simulink model "SHipVar5_OpVnesh"  (R2022a)
settings: Solver=ode23tb  StartTime=0.0  StopTime=time  MaxStep=1e-5  RelTol=1e-5
undefined symbols (not defined in the file): Imax, OpVnesh, Rd, source, U_1
libraries: spsFourierLib x2, spsDiodeLib x1, spsIGBTLib x1, simulink x1, spsSeriesRLCBranchLib x1, spsDCVoltageSourceLib x1, spsVoltageMeasurementLib x1, spsCurrentMeasurementLib x1, spspowerguiLib x1
settings Model: Creator=админ  LastModifiedBy=админ

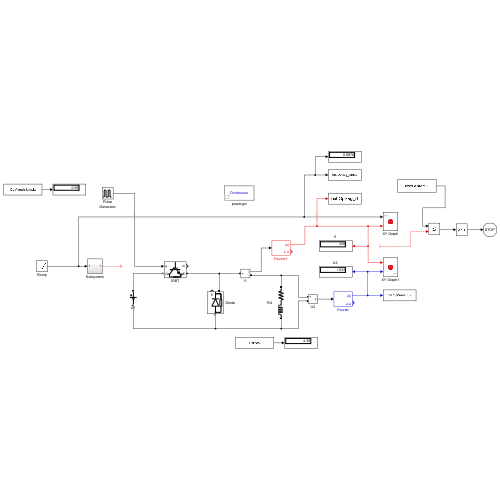
[thumbnail: Simulink's stored preview of the top-level diagram]
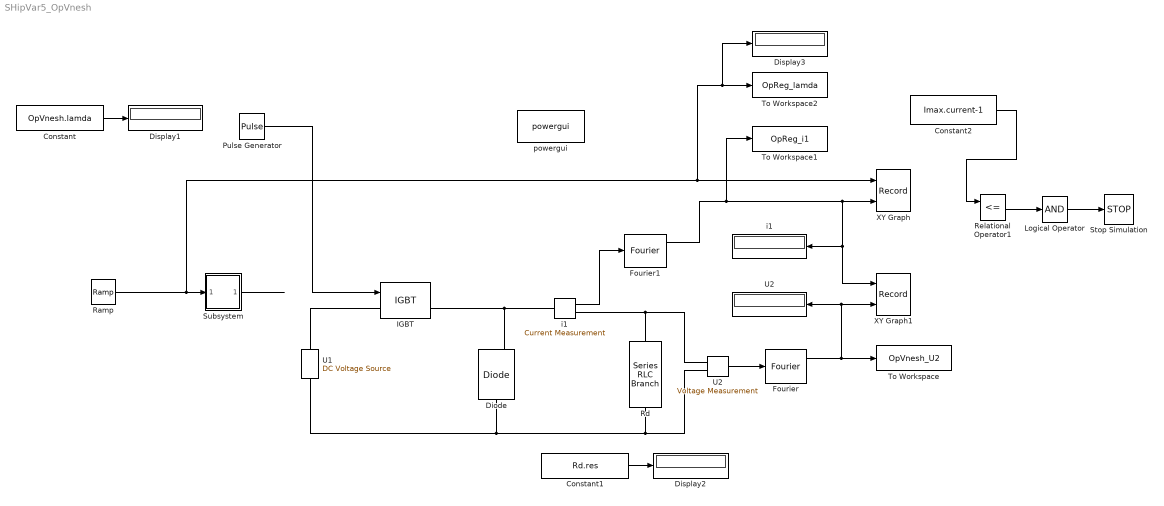
== system SHipVar5_OpVnesh ==
  Constant : Constant  Value=OpVnesh.lamda
  Constant1 : Constant  Value=Rd.res
  Constant2 : Constant  Value=Imax.current-1
  Diode : spsDiodeLib/Diode  Ron=Diode.r_t  Lon=0  Vf=0.8  IC=0  UseSnubber=0  Rs=Diode.R_s  Cs=250e-9  Measurements=on
  Display1 : Display
  Display2 : Display
  Display3 : Display
  Fourier : spsFourierLib/Fourier  Freq=source.f_c  n=0  InInit=[0, 0]  Ts=0
      settings: SourceProductBaseCode=PS
  Fourier1 : spsFourierLib/Fourier  Freq=source.f_c  n=0  InInit=[0, 0]  Ts=0
      settings: SourceProductBaseCode=PS
  IGBT : spsIGBTLib/IGBT  Ron=IGBT.R_on  Lon=0  Vf=IGBT.V_f  Tf=1e-6  Tt=2e-6  IC=0  Rs=1e5  Cs=inf  Measurements=on
  Logical Operator : Logic  Inputs=1  AllPortsSameDT=off  OutDataTypeStr=boolean
  Pulse Generator : DiscretePulseGenerator  PulseType=Time based  Period=1/source.f_c  PulseWidth=OpVnesh.lamda*100
  Ramp : simulink/Sources/Ramp  slope=0.1  start=0  InitialOutput=0
  Rd : spsSeriesRLCBranchLib/Series RLC Branch  LConnTagsString=__new0  RConnTagsString=__new0  BranchType=RL  Resistance=Rd.res  Inductance=Rd.ind  SetiL0=off  InitialCurrent=0  Capacitance=1e-6  Setx0=off  InitialVoltage=0  Measurements=None
  Relational Operator1 : RelationalOperator  Operator=<=  OutDataTypeStr=boolean  RndMeth=Simplest  InputSameDT=off
  Stop Simulation : Stop
  Subsystem : Subsystem
  To Workspace : ToWorkspace  VariableName=OpVnesh_U2  SaveFormat=Structure  SampleTime=-1
      settings: Save2DSignal=2-D array (concatenate along first dimension)
  To Workspace1 : ToWorkspace  VariableName=OpReg_i1  SaveFormat=Structure  SampleTime=-1
      settings: Save2DSignal=2-D array (concatenate along first dimension)
  To Workspace2 : ToWorkspace  VariableName=OpReg_lamda  SaveFormat=Structure  SampleTime=-1
      settings: Save2DSignal=2-D array (concatenate along first dimension)
  U1 : spsDCVoltageSourceLib/DC Voltage Source  Amplitude=U_1  Measurements=None
  U2 : spsVoltageMeasurementLib/Voltage Measurement  PhasorSimulation=off  OutputType=Complex  PSBequivalent=0
  "U2 " : Display
  XY Graph : Record  FileSettingsInternal="{\"entries\":[{\"content\":{\"excelSettings\":{\"content\":{},\"type\":\"Streamout.ExcelSettings\"}},\"type\":\"Streamout.FileSettingStorage\",\"uuid\":\"23574a75-d7b5-437e-9ab1-f31661b62460\"}],\"packageUris\":[\"http://schema.mathworks.com/mf0/streamout_blocks/R2020a\"],\"version\":\"1.0\"}"  Layout=[1 1]  SignalsInternal="{\"entries\":[{\"content\":{\"signals\":[{\"content\":{\"blockPath\":[\"SHipVar5_OpVnesh/XY Graph\"],\"channel\":[],\"dimensions\":[1],\"domain\":\"SHipVar5_OpVnesh/XY Graph\",\"lineColor\":\"#a2142f\",\"plots\":[1],\"port\":1,\"sid\":[\"\"],\"signalID\":4300,\"signalName\":\"Ramp\"},\"type\":\"RecordBlkView.Signal\",\"uuid\":\"330522d2-f3ca-434a-8d93-8c397e8adb3c\"},{\"content\":{\"blockPath\":[\"SHipVar5_OpVnesh/XY Graph\"],\"channel\":[],\"dimensions\":[1],\"domain\":\"SHipVar5_OpVnesh/XY Graph\",\"lineColor\":\"#139fff\",\"plots\":[1],\"port\":2,\"sid\":[\"\"],\"signalID\":4304,\"signalName\":\"Fourier1:1\"},\"type\":\"RecordBlkView.Signal\",\"uuid\":\"7fa0577b-ccd9-48e4-9d98-3b11980c29aa\"}]},\"type\":\"RecordBlkView.InputSignals\",\"uuid\":\"1c9948c1-7f7b-4c40-b817-17e788a1b9c1\"}],\"packageUris\":[\"http://schema.mathworks.com/mf0/streamout_blocks/R2020a\"],\"version\":\"1.0\"}"  VisualizationBindings="{\"xyplotplugin\":{\"info\":[{\"series\":[{\"bindingParametersList\":[{\"parameter\":\"X-Axis\",\"signalID\":4300,\"signalName\":\"Ramp\"},{\"parameter\":\"Y-Axis\",\"signalID\":4304,\"signalName\":\"Fourier1:1\"}],\"seriesID\":45275}],\"subplotID\":1}]}}"  CompatibilityTag=XY
  XY Graph1 : Record  FileSettingsInternal="{\"entries\":[{\"content\":{\"excelSettings\":{\"content\":{},\"type\":\"Streamout.ExcelSettings\"}},\"type\":\"Streamout.FileSettingStorage\",\"uuid\":\"e7ce2358-359a-45fa-9b79-56cba1cac5cb\"}],\"packageUris\":[\"http://schema.mathworks.com/mf0/streamout_blocks/R2020a\"],\"version\":\"1.0\"}"  Layout=[1 1]  SignalsInternal="{\"entries\":[{\"content\":{\"signals\":[{\"content\":{\"blockPath\":[\"SHipVar5_OpVnesh/XY Graph1\"],\"channel\":[],\"dimensions\":[1],\"domain\":\"SHipVar5_OpVnesh/XY Graph1\",\"lineColor\":\"#a2142f\",\"plots\":[1],\"port\":1,\"sid\":[\"\"],\"signalID\":4308,\"signalName\":\"Fourier1:1\"},\"type\":\"RecordBlkView.Signal\",\"uuid\":\"d5f5a975-f57f-42e8-bd8c-c4c1de54bcdc\"},{\"content\":{\"blockPath\":[\"SHipVar5_OpVnesh/XY Graph1\"],\"channel\":[],\"dimensions\":[1],\"domain\":\"SHipVar5_OpVnesh/XY Graph1\",\"lineColor\":\"#139fff\",\"plots\":[1],\"port\":2,\"sid\":[\"\"],\"signalID\":4312,\"signalName\":\"Fourier:1\"},\"type\":\"RecordBlkView.Signal\",\"uuid\":\"1d470808-ef71-43c9-86f4-7795574ddb1a\"}]},\"type\":\"RecordBlkView.InputSignals\",\"uuid\":\"453252bf-c3a8-49dd-a759-dd61e3aad6bf\"}],\"packageUris\":[\"http://schema.mathworks.com/mf0/streamout_blocks/R2020a\"],\"version\":\"1.0\"}"  VisualizationBindings="{\"xyplotplugin\":{\"info\":[{\"series\":[{\"bindingParametersList\":[{\"parameter\":\"X-Axis\",\"signalID\":4308,\"signalName\":\"Fourier1:1\"},{\"parameter\":\"Y-Axis\",\"signalID\":4312,\"signalName\":\"Fourier:1\"}],\"seriesID\":6124}],\"subplotID\":1}]}}"  CompatibilityTag=XY
  i1 : spsCurrentMeasurementLib/Current Measurement  PhasorSimulation=off  OutputType=Complex  PSBequivalent=0
  "i1 " : Display
  powergui : spspowerguiLib/powergui  Priority=1  SimulationMode=Continuous  SampleTime=50e-6  frequency=60  Iterations=50  frequencyindice=0  Pbase=100e6  ErrMax=1e-4  UnitsV=kV  UnitsW=MW  buscounter=0  FunctionMessages=off  echomessages=off  EnableUseOfTLC=off  CurrentSourceSwitches=off  DisableSnubberDevices=off  DisableRonSwitches=off  DisableVfSwitches=off  DisplayEquations=off  AutomaticDiscreteSolvers=off  SolverType=Tustin/Backward Euler (TBE)  Interpol=off  ExternalGateDelay=off  methode=off  Ts=100  x0status=blocks  SPID=on  SwTol=0  HookPort=off  NonlinearTolerance=1e-4  nMaxIteration=100  ContinueOnMaxIteration=off  RestoreLinks=warning  ResistiveCurrentMeasurement=off  Frange=[0:2:500]  Ylog=off  Xlog=on  ShowGrid=off  save=off  variable=ZData  structure=0  ZoomFFT=off  StartTime=0.0  cycles=1  DisplayStyle=1  fundamental=60  FreqAxis=off  MaxFrequency=1000  frequencyindicesteady=1  RmsSteady=1  display=off
  wires:
  U2/1 -> Fourier/1
  i1/1 -> Fourier1/1
  Ramp/1 -> XY Graph/1, Display3/1, To Workspace2/1, Subsystem/1(In1)
  Fourier/1 -> To Workspace/1, "U2 "/1, XY Graph1/2
  Constant/1 -> Display1/1
  Constant1/1 -> Display2/1
  Fourier1/1 -> XY Graph1/1, "i1 "/1, XY Graph/2, To Workspace1/1
  Relational Operator1/1 -> Logical Operator/1
  Constant2/1 -> Relational Operator1/1
  Logical Operator/1 -> Stop Simulation/1
  Subsystem/1(Out1) -> ?
  ? -> Relational Operator1/2
  Pulse Generator/1 -> IGBT/1
  connections:
  Diode/RConn1 -- IGBT/RConn1 -- i1/LConn1
  Rd/LConn1 -- i1/RConn1 -- U2/LConn1
  Diode/LConn1 -- U1/LConn1 -- Rd/RConn1 -- U2/LConn2
  IGBT/LConn1 -- U1/RConn1

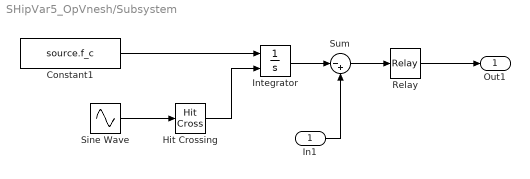
== system SHipVar5_OpVnesh/Subsystem ==
  In1 : Inport
  Constant1 : Constant  Value=source.f_c
  Hit Crossing : HitCross
  Integrator : Integrator  ExternalReset=rising
  Relay : Relay
  Sine Wave : Sin  Frequency=pi*source.f_c  SampleTime=0
  Sum : Sum  Inputs=|-+
  Out1 : Outport
  wires:
  Integrator/1 -> Sum/1
  Sum/1 -> Relay/1
  Sine Wave/1 -> Hit Crossing/1
  Hit Crossing/1 -> Integrator/2
  Constant1/1 -> Integrator/1
  In1/1 -> Sum/2
  Relay/1 -> Out1/1
